simulink model "Suspension_system"  (R2020b)
settings: Solver=VariableStepAuto  StartTime=0.0  StopTime=100  RelTol=1e-3
values from neighbouring files (symbols this model uses):
  b = 290    [Suspension_system_values.m]
  k1 = 5700    [Suspension_system_values.m]
  k2 = 135000    [Suspension_system_values.m]
  m1 = 465    [Suspension_system_values.m]
  m2 = 50    [Suspension_system_values.m]
settings Model: Creator=shubham sharma  LastModifiedBy=shubham sharma

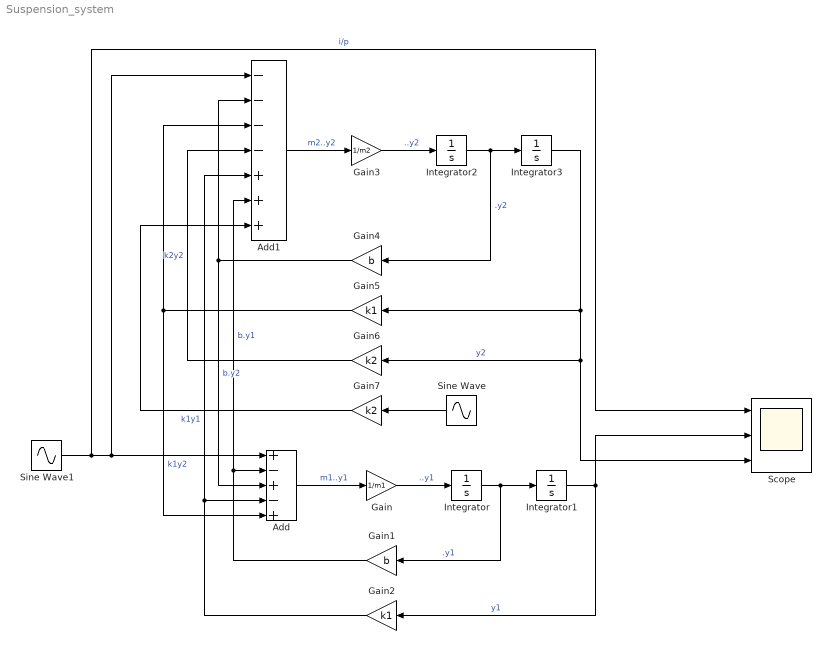
== system Suspension_system ==
  Add : Sum  Inputs=+-+-+
  Add1 : Sum  Inputs=----+++
  Gain : Gain  Gain=1/m1
  Gain1 : Gain  Gain=b
  Gain2 : Gain  Gain=k1
  Gain3 : Gain  Gain=1/m2
  Gain4 : Gain  Gain=b
  Gain5 : Gain  Gain=k1
  Gain6 : Gain  Gain=k2
  Gain7 : Gain  Gain=k2
  Integrator{,1..3} (4 alike) : Integrator
  Scope : Scope  NumInputPorts=3
  Sine Wave : Sin  SampleTime=0
  Sine Wave1 : Sin  SampleTime=0
  wires:
  Gain/1 -> Integrator/1  "..y1"
  Add/1 -> Gain/1  "m1..y1"
  Gain1/1 -> Add/2, Add1/6  "b.y1"
  Sine Wave1/1 -> Scope/1, Add1/1, Add/1  "i/p"
  Integrator/1 -> Gain1/1, Integrator1/1  ".y1"
  Integrator1/1 -> Scope/2, Gain2/1  "y1"
  Gain2/1 -> Add1/5, Add/4  "k1y1"
  Add1/1 -> Gain3/1  "m2..y2"
  Gain3/1 -> Integrator2/1  "..y2"
  Integrator2/1 -> Gain4/1, Integrator3/1  ".y2"
  Gain4/1 -> Add1/2, Add/3  "b.y2"
  Integrator3/1 -> Scope/3, Gain6/1, Gain5/1  "y2"
  Gain5/1 -> Add1/3, Add/5  "k1y2"
  Gain6/1 -> Add1/4  "k2y2"
  Sine Wave/1 -> Gain7/1
  Gain7/1 -> Add1/7
